simulink model "hdot_dele"  (R2014b)
settings: Solver=ode45  StartTime=0.0  StopTime=10.0  RelTol=1e-3
values from neighbouring files (symbols this model uses):
  A = [X_u + a * X_wdot * Z_u   X_w + a * X_wdot * Z_w   X_q + a * X_wdot * (u_0 + Z_q)   -g * (cos(theta_0) + a * X_wdot * sin(theta_0))   0 ... (first row only)    [controller_design.m]    (also in midterm.m)
  B = [a * X_wdot * Z_d_e + X_d_e   a * X_wdot * Z_d_T + X_d_T   -(X_u + a * X_wdot * Z_u) ... (first row only)    [controller_design.m]    (also in midterm.m)
  C = [1    0       0   0     0 ... (first row only)    [controller_design.m]    (also in midterm.m)
  D = [0   0   0 ... (first row only)    [controller_design.m]    (also in midterm.m)
  ugstep = -20    [midterm.m]
settings Model: Creator=karasinski  LastModifiedBy=karasinski

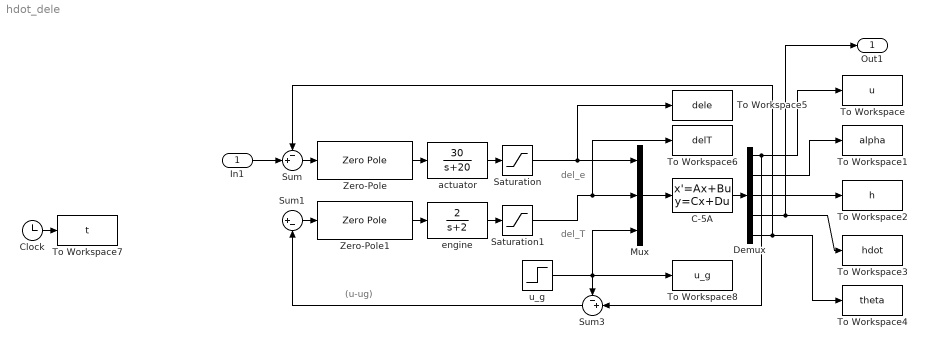
== system hdot_dele ==
  note: del_e
  note: del_T
  note: (u-ug)
  In1 : Inport
  C-5A : StateSpace  A=A  B=B  C=C  D=D  X0=0
  Clock : Clock
  Demux : Demux  Outputs=5
  Mux : Mux  Inputs=3
  Saturation : Saturate  UpperLimit=20/57.3  LowerLimit=-20/57.3
  Saturation1 : Saturate  UpperLimit=70000  LowerLimit=-70000
  Sum : Sum  Inputs=-+|
  Sum1 : Sum  Inputs=|+-
  Sum3 : Sum  Inputs=-+|
  To Workspace : ToWorkspace  VariableName=u  SampleTime=-1
  To Workspace1 : ToWorkspace  VariableName=alpha  SampleTime=-1
  To Workspace2 : ToWorkspace  VariableName=h  SampleTime=-1
  To Workspace3 : ToWorkspace  VariableName=hdot  SampleTime=-1
  To Workspace4 : ToWorkspace  VariableName=theta  SampleTime=-1
  To Workspace5 : ToWorkspace  VariableName=dele  SampleTime=-1
  To Workspace6 : ToWorkspace  VariableName=delT  SampleTime=-1
  To Workspace7 : ToWorkspace  VariableName=t  SampleTime=-1
  To Workspace8 : ToWorkspace  VariableName=u_g  SampleTime=-1
  Zero-Pole : ZeroPole  Zeros=[-.8 -.1]  Poles=[0 -2 -100]  Gain=[-260]
  Zero-Pole1 : ZeroPole  Zeros=[-.1]  Poles=[0 -5]  Gain=[30909]
  actuator : TransferFcn  Numerator=[30]  Denominator=[1 20]
  engine : TransferFcn  Numerator=[2]  Denominator=[1 2]
  u_g : Step  Time=0  After=ugstep  SampleTime=0
  Out1 : Outport
  wires:
  Mux/1 -> C-5A/1
  C-5A/1 -> Demux/1
  actuator/1 -> Saturation/1
  Demux/1 -> To Workspace/1, Sum3/2
  Demux/2 -> To Workspace1/1
  Demux/3 -> To Workspace2/1
  Demux/4 -> Out1/1, To Workspace3/1
  Demux/5 -> To Workspace4/1, Sum/1
  Clock/1 -> To Workspace7/1
  engine/1 -> Saturation1/1
  Zero-Pole/1 -> actuator/1
  Zero-Pole1/1 -> engine/1
  Sum1/1 -> Zero-Pole1/1
  Sum3/1 -> Sum1/2
  Sum/1 -> Zero-Pole/1
  In1/1 -> Sum/2
  Saturation/1 -> Mux/1, To Workspace5/1
  Saturation1/1 -> Mux/2, To Workspace6/1
  u_g/1 -> Mux/3, To Workspace8/1, Sum3/1
